simulink model "E_Platoon_simscape"  (R2025b)
settings: Solver=FixedStepAuto  StartTime=0.0  StopTime=inf  FixedStep=0.01  RelTol=1e-3
values from neighbouring files (symbols this model uses):
  battery_SOC_resistance = battery_SOC(:,3)    [EV_Truck.m]
  battery_SOC_SOC = battery_SOC(:,1)    [EV_Truck.m]
  battery_SOC_voltage = battery_SOC(:,2)    [EV_Truck.m]
  motor_efficiency_efficiency = table2array(motor_efficiency(2:height(motor_efficiency),2:width(motor_efficiency)))    [EV_Truck.m]
  motor_efficiency_RPM = table2array(motor_efficiency(2:height(motor_efficiency),1))    [EV_Truck.m]
  motor_efficiency_torque = transpose(motor_efficiency_torque)    [EV_Truck.m]
  motor_RPM_torque = table2array(motor_torque(1:14,1))    [EV_Truck.m]
  motor_torque_RPM = table2array(motor_torque(1:14,2))    [EV_Truck.m]
undefined symbols (not defined in the file or in its folder): battery_builder_rtmsupport, DiscIntNeverNeededParam, gcbh
libraries: simulink x8, fl_lib x8, nesl_utility x8, Batteries_lib x4, mpcadaslib x2, slpidlib x2
(part 2 of 3)

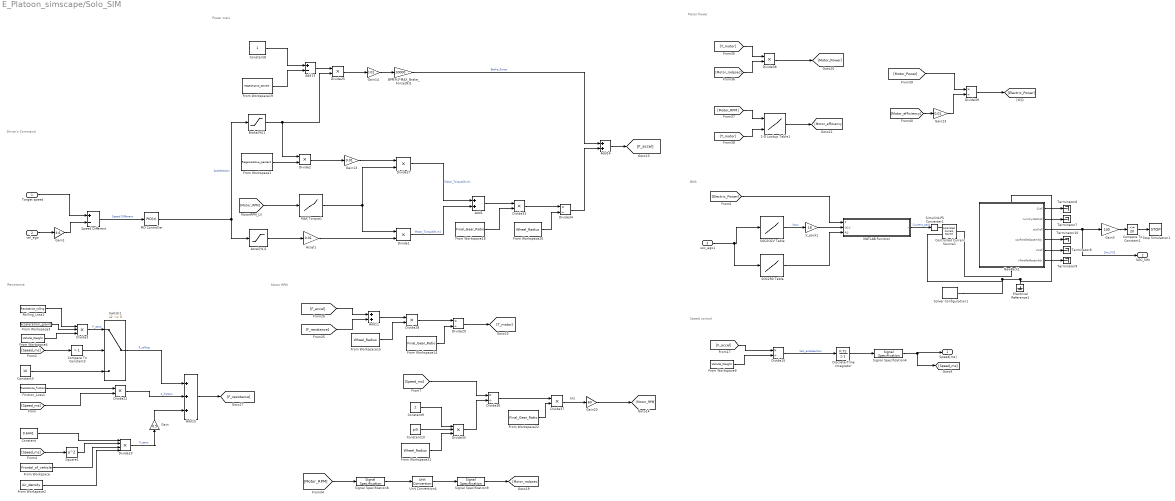
== system E_Platoon_simscape/Solo_SIM ==
  note: Speed control
  note: Driver's Command
  note: RPS
  note: Power train
  note: Resistance
  note: Motor RPM
  note: Motor Power
  note: BMS
  Target speed : Inport
  vel_ego : Inport  Port=2
  soc_ego1 : Inport  Port=3
  2-D Lookup Table1 : Lookup_n-D  BreakpointsForDimension1=motor_efficiency_RPM  BreakpointsForDimension2=motor_efficiency_torque  Table=motor_efficiency_efficiency  InternalRulePriority=Speed  RndMeth=Simplest
      settings: InputPortMap=u0,u1
  Accel1 : Gain  Gain=0.01
  Accel[%]1 : Saturate  UpperLimit=100  LowerLimit=0
  Add1 : Sum
  Add11 : Sum
  Add13 : Sum  Inputs=+-
  Add14 : Sum
  Add15 : Sum  Inputs=+++
  BPP[%]*MAX_Brake_Force[N]1 : Gain  Gain=10000
  Brake[%]1 : Saturate  UpperLimit=0  LowerLimit=-100
  Compare To Constant1 : simulink/Logic and Bit Operations/Compare To Constant  relop=<=  const=20  OutDataTypeStr=boolean
  Compare To Constant3 : simulink/Logic and Bit Operations/Compare To Constant  relop=>  const=1  OutDataTypeStr=boolean
  Constant : Constant  Value=0.6441
  Constant10 : Constant  Value=pi()
  Constant3 : Constant  Value=10
  Constant8 : Constant
  Constant9 : Constant  Value=2
  Controlled Current Source1 : fl_lib/Electrical/Electrical Sources/Controlled Current Source
  Discrete-Time Integrator : DiscreteIntegrator  SampleTime=-1  ICPrevOutput=DiscIntNeverNeededParam  ICPrevScaledInput=DiscIntNeverNeededParam
  Divide{1..2,22,25,27..28,33,37..38} (9 alike) : Product  Inputs=**
  Divide{15,29,34,36,39} (5 alike) : Product  Inputs=*/
  Divide23 : Product  Inputs=****
  Divide3 : Product  Inputs=***
  Divide35 : Product  Inputs=***
  Electrical Reference1 : fl_lib/Electrical/Electrical Elements/Electrical Reference
  Friction_Loss1 : FromWorkspace  VariableName=Resistance_friction  SampleTime=0.01
  From Workspace : FromWorkspace  VariableName=Frontal_of_vehicle  SampleTime=0.01
  From Workspace1 : FromWorkspace  VariableName=Regenerative_percent  SampleTime=0.01
  From Workspace14 : FromWorkspace  VariableName=Final_Gear_Ratio  SampleTime=0.01
  From Workspace15 : FromWorkspace  VariableName=Wheel_Radius  SampleTime=0.01
  From Workspace18 : FromWorkspace  VariableName=Final_Gear_Ratio  SampleTime=0.01
  From Workspace19 : FromWorkspace  VariableName=Regenerative_percent  SampleTime=0.01
  From Workspace2 : FromWorkspace  VariableName=Air_density  SampleTime=0.01
  From Workspace20 : FromWorkspace  VariableName=Wheel_Radius  SampleTime=0.01
  From Workspace21 : FromWorkspace  VariableName=Wheel_Radius  SampleTime=0.01
  From Workspace22 : FromWorkspace  VariableName=Final_Gear_Ratio  SampleTime=0.01
  From Workspace3 : FromWorkspace  VariableName=Acceleration_gravity  SampleTime=0.01
  From Workspace4 : FromWorkspace  VariableName=Vehicle_Weight  SampleTime=0.01
  From Workspace9 : FromWorkspace  VariableName=Vehicle_Weight  SampleTime=0.01
  Gain : Gain  Gain=0.5
  Gain1 : Gain  Gain=3.6
  Gain13 : Gain  Gain=0.01
  Gain14 : Gain  Gain=0.01
  Gain20 : Gain  Gain=60
  Gain23 : Gain  Gain=0.01
  Gain3 : Gain  Gain=100
  MATLAB Function : MATLAB Function  TreatAsAtomicUnit=on
  MAX Torque1 : Lookup_n-D  NumberOfTableDimensions=1  BreakpointsForDimension1=motor_RPM_torque  Table=motor_torque_RPM  InternalRulePriority=Speed  RndMeth=Simplest
  NewPack1 : Subsystem  LoadFcn=battery_builder_rtmsupport('loadfcn',gcbh);
      settings: CopyFcn=battery_builder_rtmsupport('copyfcn',gcbh);  PreCopyFcn=battery_builder_rtmsupport('precopyfcn',gcbh);  PreDeleteFcn=battery_builder_rtmsupport('predeletefcn',gcbh);  PortSchema="{\"entries\":[{\"content\":{\"sides\":[{\"content\":{\"connectorIds\":[\"LConn1\"]},\"type\":\"ConnectorPlacement.EquallySpacedRectSide\",\"uuid\":\"1202e0a0-be56-4819-949f-0e575ff0fad5\"},{\"content\":{\"connectorIds\":[\"RConn1\"],\"side\":\"RIGHT\"},\"type\":\"ConnectorPlacement.EquallySpacedRectSide\",\"uuid\":\"c846b010-7318-4529-a495-49262266c279\"},{\"content\":{\"side\":\"TOP\"},\"type\":\"ConnectorPlacement.EquallySpacedRectSide\",\"uuid\":\"5cadc0b8-a7f2-47b4-97e8-4fab1bc2ac7d\"},{\"content\":{\"connectorIds\":[\"Out1\",\"Out2\",\"Out3\",\"Out4\",\"Out5\",\"Out6\"],\"side\":\"BOTTOM\"},\"type\":\"ConnectorPlacement.EquallySpacedRectSide\",\"uuid\":\"c5ce92ef-d0c0-4ddc-9166-c3c67527b5cc\"}]},\"type\":\"ConnectorPlacement.EquallySpacedConnector\",\"uuid\":\"4d056c7c-5936-459e-9daf-456b1978dca2\"}],\"packageUris\":[\"http://schema.mathworks.com/mf0/Connector/R2020b\"],\"version\":\"1.0\"}"
      mask Display: image('$imagefile')
  PID Controller : slpidlib/PID Controller  Controller=PID  Form=Parallel  TimeDomain=Discrete-time  UseExternalTs=off  SampleTime=0.01  IntegratorMethod=Forward Euler  FilterMethod=Forward Euler  ControllerParametersSource=internal  P=100  I=0.01  UseKiTs=off  D=0.0001  UseExternalDerivativeSource=off  N=10  UseFilter=on  TunerSelectOption=Transfer Function Based (PID Tuner App)  InitialConditionSource=internal  InitialConditionForIntegrator=0  InitialConditionForFilter=0  DifferentiatorICPrevScaledInput=0  ExternalReset=none  TrackingMode=off  Kt=1  LimitOutput=off  SatLimitsSource=internal  UpperSaturationLimit=inf  LowerSaturationLimit=-inf  LinearizeAsGain=on  AntiWindupMode=none  Kb=1  LimitIntegrator=off  UpperIntegratorSaturationLimit=inf  LowerIntegratorSaturationLimit=-inf  POutMin=[]  POutMax=[]  IOutMin=[]  IOutMax=[]  DOutMin=[]  DOutMax=[]  NOutMin=[]  NOutMax=[]  SumOutMin=[]  SumOutMax=[]  SaturationOutMin=[]  SaturationOutMax=[]  PParamMin=[]  PParamMax=[]  IParamMin=[]  IParamMax=[]  DParamMin=[]  DParamMax=[]  NParamMin=[]  NParamMax=[]  KbParamMin=[]  KbParamMax=[]  KtParamMin=[]  KtParamMax=[]  KbOutMin=[]  KbOutMax=[]  KtOutMin=[]  KtOutMax=[]  IntegratorOutMin=[]  IntegratorOutMax=[]  FilterOutMin=[]  FilterOutMax=[]  SumI1OutMin=[]  SumI1OutMax=[]  SumI2OutMin=[]  SumI2OutMax=[]  SumI3OutMin=[]  SumI3OutMax=[]  SumI4OutMin=[]  SumI4OutMax=[]  SumDOutMin=[]  SumDOutMax=[]  DifferentiatorOutMin=[]  DifferentiatorOutMax=[]  FilterDiffOutCoefMin=[]  FilterDiffOutCoefMax=[]  ReciprocalOutMin=[]  ReciprocalOutMax=[]  SumDenOutMin=[]  SumDenOutMax=[]  SumNumOutMin=[]  SumNumOutMax=[]  DivideOutMin=[]  DivideOutMax=[]  UdiffTsProdOutMin=[]  UdiffTsProdOutMax=[]  NTsProdOutMin=[]  NTsProdOutMax=[]  UintegralTsProdOutMin=[]  UintegralTsProdOutMax=[]  UngainTsProdOutMin=[]  UngainTsProdOutMax=[]  ClampingZeroOutDataTypeStr=Inherit: Inherit via back propagation  ClampingZeroOutMin=[]  ClampingZeroOutMax=[]  FilterDenConstantOutDataTypeStr=Inherit: Inherit via back propagation  FilterDenConstantOutMin=[]  FilterDenConstantOutMax=[]  PCopyOutDataTypeStr=Inherit: Inherit via back propagation  PCopyOutMin=[]  PCopyOutMax=[]  NCopyOutDataTypeStr=Inherit: Inherit via back propagation  NCopyOutMin=[]  NCopyOutMax=[]  IntegratorContinuousStateAttributes=''  IntegratorStateMustResolveToSignalObject=off  IntegratorRTWStateStorageClass=Auto  FilterContinuousStateAttributes=''  FilterStateMustResolveToSignalObject=off  FilterRTWStateStorageClass=Auto  ParallelPVariant=InternalParameters  IdealPVariant=Disabled  IVariant=InternalParameters  DVariant=InternalParameters  IntegratorVariant=Discrete  SatVariant=Disabled  AWVariant=Passthrough  PCopyVariant=Disabled  TRVariant=Disabled  FdbkBlocksVariant=Forward  IdealPFdbkVariant=Disabled  SatFdbkVariant=Disabled  DerivativeFilterVariant=ForwardEulerFilter  NVariant=InternalParameters  NCopyVariant=Disabled  FilterICVariant=InternalICsFilter  IntegratorICVariant=InternalICs  ExternalResetVariant=Disabled  TRSumVariant=Passthrough  SumFdbkVariant=Disabled  SumVariant=Sum_PID  TsampFilterVariant=InternalTs  TsampNgainVariant=Passthrough  TsampIntegralVariant=Disabled_SignalSpec  ExternalSaturationOutDataTypeStr=Inherit: Same as second input  DerivativeSourceVariant=ErrorSignal  PreIntVariant=InternalPreInt
  Rolling_Loss1 : FromWorkspace  VariableName=Resistance_rolling  SampleTime=0.01
  SOC2OCV Table : Lookup_n-D  NumberOfTableDimensions=1  BreakpointsForDimension1=battery_SOC_SOC  Table=battery_SOC_voltage  ExtrapMethod=Clip  RemoveProtectionInput=on  UseLastTableValue=on  InternalRulePriority=Speed  RndMeth=Simplest
  SOC2R0 Table : Lookup_n-D  NumberOfTableDimensions=1  BreakpointsForDimension1=battery_SOC_SOC  Table=battery_SOC_resistance  RemoveProtectionInput=on  InternalRulePriority=Speed  RndMeth=Simplest
  Signal Specification4 : SignalSpecification  Unit=m/s
  Signal Specification8 : SignalSpecification  Unit=rpm
  Signal Specification9 : SignalSpecification  Unit=rad/s
  Simulink-PS Converter1 : nesl_utility/Simulink-PS Converter  PhysicalDomain=network_engine_domain  SubClassName=ps_input  LeftPortType=input  RightPortType=output  PseudoPeriodic=off  Frequencies=[]  NoiseDistribution=none  NoiseParameters=[]  Unit=1  AffineConversion=off  FilteringAndDerivatives=provide  SimscapeFilterOrder=1  InputFilterTimeConstant=0.001  UdotUserProvided=0
  Solver Configuration1 : nesl_utility/Solver Configuration  PhysicalDomain=network_engine_domain  SubClassName=solver  LeftPortType=input  RightPortType=generic  Tones=[]  Harmonics=[]  SimulateNoise=off  Profile=off  UseLocalSampling=off  EnableSwitchedLinearOptims=on  FrequencyDomain=off  UseCCode=off  RelTol=0.001  AbsTol=0.001  MinStep=1e-09  ToWorkspace=off  RevertToSquareIcSolve=off  NumHomotopyIterations=100  PhasorMode=off  PhasorModeNumHarmonics=1  ConsistencySolver=NEWTON_XTOL_AFTER_FTOL  IndexReductionMethod=DerivativeReplacement  DoDC=on  ResidualTolerance=1e-09  ConsistencyTolSource=GLOBAL  ConsistencyAbsTol=0.001  ConsistencyRelTol=0.001  ConsistencyTolFactor=0.001  UseLocalSolver=off  LocalSolverChoice=NE_BACKWARD_EULER_ADVANCER  ResolveIndetEquations=on  FunctionEvalNumThread=1  LocalSolverSampleTime=0.01  DoFixedCost=off  MaxNonlinIter=3  MaxModeIter=2  ComputeImpulses=off  ImpulseIterations=2  LinearAlgebra=auto  LinearAlgebraNumThread=0  EquationFormulation=NE_TIME_EF  DelaysMemoryBudget=1024  AutomaticFiltering=on  FilteringTimeConstant=0.001  PartitionStorageMethod=AS_NEEDED  PartitionMemoryBudget=1024  PartitionMethod=ROBUST  MultibodyUseLocalSolver=off  MultibodyLocalSolverChoice=ODE1  MultibodyLocalSolverSampleTime=0.001
  Speed Different : Sum  Inputs=+-
  Square1 : Math  Operator=square
  Stop Simulation1 : Stop
  Switch1 : Switch  Criteria=u2 ~= 0  SaturateOnIntegerOverflow=off  InputSameDT=off
  Terminator{6..10} (5 alike) : Terminator
  Unit Conversion4 : UnitConversion
  V_pack1 : Gain  Gain=18
  Speed[ms] : Outport
  SOC_SIM : Outport  Port=2
  wires:
  From Workspace9/1 -> Divide15/2
  Divide15/1 -> Discrete-Time Integrator/1  "Veh_acceleartion"
  Discrete-Time Integrator/1 -> Signal Specification4/1
  Signal Specification4/1 -> Speed[ms]/1, [Speed_ms]
  PID Controller/1 -> Brake[%]1/1, Accel[%]1/1  "Acceleration"
  Speed Different/1 -> PID Controller/1  "Speed Different"
  Target speed/1 -> Speed Different/1
  vel_ego/1 -> Gain1/1
  Divide28/1 -> Divide29/1
  From Workspace20/1 -> Divide34/2
  Add1/1 -> Divide33/1
  [T_motor] -> Divide38/1
  Divide29/1 -> [T_motor]
  Signal Specification9/1 -> [Motor_radpsec]
  Gain20/1 -> [Motor_RPM]
  Add13/1 -> Divide25/1
  Divide39/1 -> [Electric_Power]
  Add14/1 -> [F_accel]
  [Speed_ms] -> Divide22/2
  [F_resistance] -> Add11/2
  Divide1/1 -> Add1/2  "Motor_Torque[N.m]"
  From Workspace14/1 -> Divide29/2
  Divide23/1 -> Gain/1  "F_aero"
  Brake[%]1/1 -> Divide25/2, Divide2/1
  Unit Conversion4/1 -> Signal Specification9/1
  From Workspace21/1 -> Divide35/3
  Divide35/1 -> Divide36/2
  [Motor_RPM] -> 2-D Lookup Table1/1
  Gain23/1 -> Divide39/2
  Compare To Constant3/1 -> Switch1/2
  Divide37/1 -> Gain20/1
  Divide34/1 -> Add14/2
  BPP[%]*MAX_Brake_Force[N]1/1 -> Add14/1  "Brake_Force"
  From Workspace/1 -> Divide23/3
  From Workspace22/1 -> Divide37/2
  Constant9/1 -> Divide35/1
  [Motor_efficiency] -> Gain23/1
  Constant10/1 -> Divide35/2
  [Speed_ms] -> Square1/1
  Add11/1 -> Divide28/1
  Square1/1 -> Divide23/2
  2-D Lookup Table1/1 -> [Motor_efficiency]
  Gain14/1 -> BPP[%]*MAX_Brake_Force[N]1/1
  From Workspace19/1 -> Add13/2
  Add15/1 -> [F_resistance]
  Friction_Loss1/1 -> Divide22/1
  [Motor_RPM] -> Signal Specification8/1
  [Motor_radpsec] -> Divide38/2
  From Workspace1/1 -> Divide2/2
  Accel[%]1/1 -> Accel1/1
  Constant8/1 -> Add13/1
  Divide36/1 -> Divide37/1
  [Motor_Power] -> Divide39/1
  MAX Torque1/1 -> Divide27/2, Divide1/1
  Accel1/1 -> Divide1/2
  Divide33/1 -> Divide34/1
  [F_accel] -> Add11/1
  [T_motor] -> 2-D Lookup Table1/2
  Rolling_Loss1/1 -> Divide3/1
  Divide27/1 -> Add1/1  "Motor_Torque[N.m]"
  Switch1/1 -> Add15/1  "F_rolling"
  From Workspace15/1 -> Divide28/2
  Gain13/1 -> Divide27/1
  Constant3/1 -> Switch1/3
  Divide25/1 -> Gain14/1
  Divide22/1 -> Add15/2  "F_friction"
  Divide2/1 -> Gain13/1
  Divide38/1 -> [Motor_Power]
  [Motor_RPM] -> MAX Torque1/1
  Signal Specification8/1 -> Unit Conversion4/1
  From Workspace18/1 -> Divide33/2
  [Speed_ms] -> Divide36/1
  [F_accel] -> Divide15/1
  [Speed_ms] -> Compare To Constant3/1
  Gain/1 -> Add15/3
  From Workspace2/1 -> Divide23/4
  From Workspace3/1 -> Divide3/2
  From Workspace4/1 -> Divide3/3
  Divide3/1 -> Switch1/1  "F_aero"
  Gain1/1 -> Speed Different/2
  Constant/1 -> Divide23/1
  SOC2R0 Table/1 -> MATLAB Function/3(R0)
  MATLAB Function/1(I) -> Simulink-PS Converter1/1  "Current_pack"
  Compare To Constant1/1 -> Stop Simulation1/1
  soc_ego1/1 -> SOC2R0 Table/1, SOC2OCV Table/1
  [Electric_Power] -> MATLAB Function/1(P)
  NewPack1/6(vParallelAssembly) -> Terminator9/1
  NewPack1/4(socParallelAssembly) -> Terminator10/1
  NewPack1/3(socCell) -> SOC_SIM/1, Gain3/1  "Sim_FV2"
  V_pack1/1 -> MATLAB Function/2(OCV)
  NewPack1/2(numCyclesCell) -> Terminator7/1
  SOC2OCV Table/1 -> V_pack1/1  "Vsoc"
  NewPack1/1(iCell) -> Terminator6/1
  NewPack1/5(vCell) -> Terminator8/1
  Gain3/1 -> Compare To Constant1/1
  connections:
  Electrical Reference1/LConn1 -- NewPack1/LConn1 -- Controlled Current Source1/RConn2 -- Solver Configuration1/RConn1
  NewPack1/RConn1 -- Controlled Current Source1/LConn1
  Simulink-PS Converter1/RConn1 -- Controlled Current Source1/RConn1

== system E_Platoon_simscape/FV1_SIM/ACC system ==
  vel_front : Inport
  pos_front : Inport  Port=2
  vel_ego : Inport  Port=3
  pos_ego : Inport  Port=4
  Adaptive Cruise Control System : mpcadaslib/Adaptive Cruise Control System  EgoModel=tf(1,[0.5,1,0])  InitialEgoVelocity=20  DefaultSpacing=20  MaxVelocity=30  MinAcceleration=-3  amin_ext=off  MaxAcceleration=3  amax_ext=off  Ts=0.01  PredictionHorizon=100  ControllerBehavior=0.7  suboptimal=off  maxiter=10  datatypeopt=double  optmode=off  trackmode=off
  MATLAB Function : MATLAB Function  TreatAsAtomicUnit=on
  Sum : Sum  Inputs=|+-
  Sum1 : Sum  Inputs=|-+
  t_gap(s) : Constant  Value=0.5
  velocity(m/s) : Constant  Value=30
  Acceleration : Outport
  Relative Distance : Outport  Port=2
  wires:
  t_gap(s)/1 -> Adaptive Cruise Control System/2
  Sum/1 -> Relative Distance/1, Adaptive Cruise Control System/4
  Sum1/1 -> Adaptive Cruise Control System/5
  velocity(m/s)/1 -> Adaptive Cruise Control System/1
  Adaptive Cruise Control System/1 -> MATLAB Function/1(accel)
  pos_front/1 -> Sum/1
  pos_ego/1 -> Sum/2
  vel_front/1 -> Sum1/2
  vel_ego/1 -> Sum1/1, Adaptive Cruise Control System/3
  MATLAB Function/1(acceleration) -> Acceleration/1

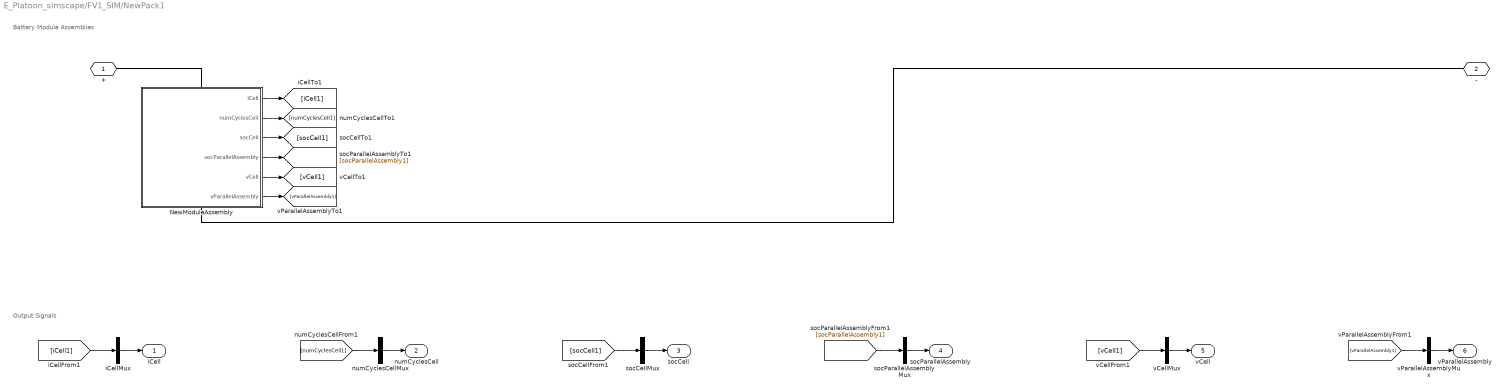
== system E_Platoon_simscape/FV1_SIM/NewPack1 ==
  note: Battery Module Assemblies
  note: Output Signals
  NewModuleAssembly : Subsystem  LoadFcn=battery_builder_rtmsupport('loadfcn',gcbh);
      settings: CopyFcn=battery_builder_rtmsupport('copyfcn',gcbh);  PreCopyFcn=battery_builder_rtmsupport('precopyfcn',gcbh);  PreDeleteFcn=battery_builder_rtmsupport('predeletefcn',gcbh);  PortSchema="{\"entries\":[{\"content\":{\"sides\":[{\"content\":{\"connectorIds\":[\"LConn1\"]},\"type\":\"ConnectorPlacement.EquallySpacedRectSide\",\"uuid\":\"1202e0a0-be56-4819-949f-0e575ff0fad5\"},{\"content\":{\"connectorIds\":[\"RConn1\"],\"side\":\"RIGHT\"},\"type\":\"ConnectorPlacement.EquallySpacedRectSide\",\"uuid\":\"c846b010-7318-4529-a495-49262266c279\"},{\"content\":{\"side\":\"TOP\"},\"type\":\"ConnectorPlacement.EquallySpacedRectSide\",\"uuid\":\"5cadc0b8-a7f2-47b4-97e8-4fab1bc2ac7d\"},{\"content\":{\"connectorIds\":[\"Out1\",\"Out2\",\"Out3\",\"Out4\",\"Out5\",\"Out6\"],\"side\":\"BOTTOM\"},\"type\":\"ConnectorPlacement.EquallySpacedRectSide\",\"uuid\":\"9f2ef959-f133-4a8d-a7c5-293375a4069f\"}]},\"type\":\"ConnectorPlacement.EquallySpacedConnector\",\"uuid\":\"4d056c7c-5936-459e-9daf-456b1978dca2\"}],\"packageUris\":[\"http://schema.mathworks.com/mf0/Connector/R2020b\"],\"version\":\"1.0\"}"
      mask Display: image('$imagefile')
  iCellMux : Mux  Inputs=1
  numCyclesCellMux : Mux  Inputs=1
  socCellMux : Mux  Inputs=1
  socParallelAssemblyMux : Mux  Inputs=1
  vCellMux : Mux  Inputs=1
  vParallelAssemblyMux : Mux  Inputs=1
  + : PMIOPort  Side=Left
  - : PMIOPort  Port=2  Side=Right
  iCell : Outport
  numCyclesCell : Outport  Port=2
  socCell : Outport  Port=3
  socParallelAssembly : Outport  Port=4
  vCell : Outport  Port=5
  vParallelAssembly : Outport  Port=6
  wires:
  NewModuleAssembly/1(iCell) -> [iCell1]
  iCellMux/1 -> iCell/1
  [iCell1] -> iCellMux/1
  NewModuleAssembly/2(numCyclesCell) -> [numCyclesCell1]
  numCyclesCellMux/1 -> numCyclesCell/1
  [numCyclesCell1] -> numCyclesCellMux/1
  NewModuleAssembly/3(socCell) -> [socCell1]
  socCellMux/1 -> socCell/1
  [socCell1] -> socCellMux/1
  NewModuleAssembly/4(socParallelAssembly) -> [socParallelAssembly1]
  socParallelAssemblyMux/1 -> socParallelAssembly/1
  [socParallelAssembly1] -> socParallelAssemblyMux/1
  NewModuleAssembly/5(vCell) -> [vCell1]
  vCellMux/1 -> vCell/1
  [vCell1] -> vCellMux/1
  NewModuleAssembly/6(vParallelAssembly) -> [vParallelAssembly1]
  vParallelAssemblyMux/1 -> vParallelAssembly/1
  [vParallelAssembly1] -> vParallelAssemblyMux/1
  connections:
  NewModuleAssembly/LConn1 -- +/RConn1
  NewModuleAssembly/RConn1 -- -/RConn1

== system E_Platoon_simscape/FV2_SIM/ACC system ==
  vel_front : Inport
  pos_front : Inport  Port=2
  vel_ego : Inport  Port=3
  pos_ego : Inport  Port=4
  Adaptive Cruise Control System : mpcadaslib/Adaptive Cruise Control System  EgoModel=tf(1,[0.5,1,0])  InitialEgoVelocity=20  DefaultSpacing=20  MaxVelocity=30  MinAcceleration=-3  amin_ext=off  MaxAcceleration=3  amax_ext=off  Ts=0.01  PredictionHorizon=100  ControllerBehavior=0.7  suboptimal=off  maxiter=10  datatypeopt=double  optmode=off  trackmode=off
  MATLAB Function : MATLAB Function  TreatAsAtomicUnit=on
  Sum : Sum  Inputs=|+-
  Sum1 : Sum  Inputs=|-+
  t_gap(s) : Constant  Value=0.5
  velocity(m/s) : Constant  Value=30
  Acceleration : Outport
  Relative Distance : Outport  Port=2
  wires:
  t_gap(s)/1 -> Adaptive Cruise Control System/2
  Sum/1 -> Relative Distance/1, Adaptive Cruise Control System/4
  Sum1/1 -> Adaptive Cruise Control System/5
  velocity(m/s)/1 -> Adaptive Cruise Control System/1
  Adaptive Cruise Control System/1 -> MATLAB Function/1(accel)
  pos_front/1 -> Sum/1
  pos_ego/1 -> Sum/2
  vel_front/1 -> Sum1/2
  vel_ego/1 -> Sum1/1, Adaptive Cruise Control System/3
  MATLAB Function/1(acceleration) -> Acceleration/1

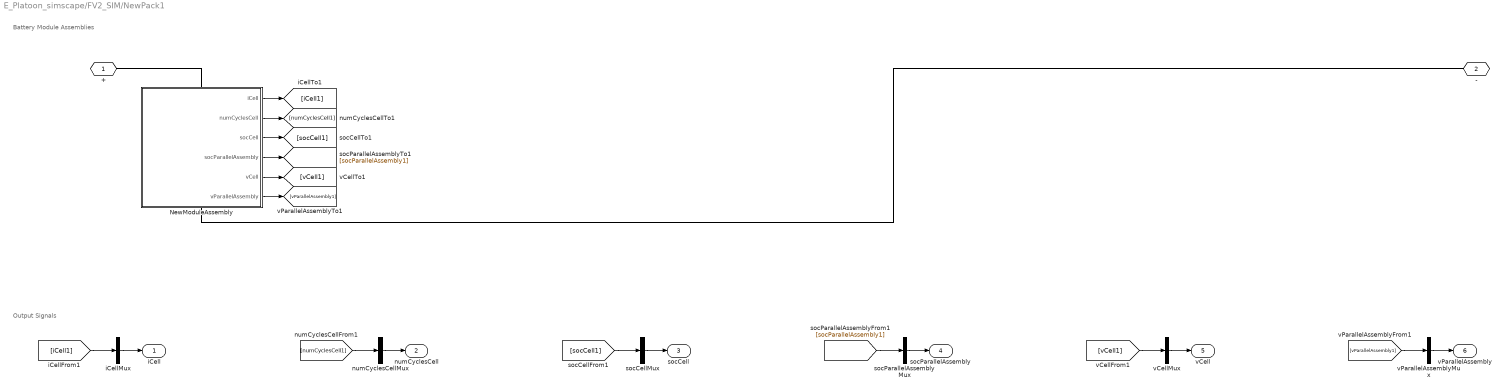
== system E_Platoon_simscape/FV2_SIM/NewPack1 ==
  note: Battery Module Assemblies
  note: Output Signals
  NewModuleAssembly : Subsystem  LoadFcn=battery_builder_rtmsupport('loadfcn',gcbh);
      settings: CopyFcn=battery_builder_rtmsupport('copyfcn',gcbh);  PreCopyFcn=battery_builder_rtmsupport('precopyfcn',gcbh);  PreDeleteFcn=battery_builder_rtmsupport('predeletefcn',gcbh);  PortSchema="{\"entries\":[{\"content\":{\"sides\":[{\"content\":{\"connectorIds\":[\"LConn1\"]},\"type\":\"ConnectorPlacement.EquallySpacedRectSide\",\"uuid\":\"1202e0a0-be56-4819-949f-0e575ff0fad5\"},{\"content\":{\"connectorIds\":[\"RConn1\"],\"side\":\"RIGHT\"},\"type\":\"ConnectorPlacement.EquallySpacedRectSide\",\"uuid\":\"c846b010-7318-4529-a495-49262266c279\"},{\"content\":{\"side\":\"TOP\"},\"type\":\"ConnectorPlacement.EquallySpacedRectSide\",\"uuid\":\"5cadc0b8-a7f2-47b4-97e8-4fab1bc2ac7d\"},{\"content\":{\"connectorIds\":[\"Out1\",\"Out2\",\"Out3\",\"Out4\",\"Out5\",\"Out6\"],\"side\":\"BOTTOM\"},\"type\":\"ConnectorPlacement.EquallySpacedRectSide\",\"uuid\":\"9f2ef959-f133-4a8d-a7c5-293375a4069f\"}]},\"type\":\"ConnectorPlacement.EquallySpacedConnector\",\"uuid\":\"4d056c7c-5936-459e-9daf-456b1978dca2\"}],\"packageUris\":[\"http://schema.mathworks.com/mf0/Connector/R2020b\"],\"version\":\"1.0\"}"
      mask Display: image('$imagefile')
  iCellMux : Mux  Inputs=1
  numCyclesCellMux : Mux  Inputs=1
  socCellMux : Mux  Inputs=1
  socParallelAssemblyMux : Mux  Inputs=1
  vCellMux : Mux  Inputs=1
  vParallelAssemblyMux : Mux  Inputs=1
  + : PMIOPort  Side=Left
  - : PMIOPort  Port=2  Side=Right
  iCell : Outport
  numCyclesCell : Outport  Port=2
  socCell : Outport  Port=3
  socParallelAssembly : Outport  Port=4
  vCell : Outport  Port=5
  vParallelAssembly : Outport  Port=6
  wires:
  NewModuleAssembly/1(iCell) -> [iCell1]
  iCellMux/1 -> iCell/1
  [iCell1] -> iCellMux/1
  NewModuleAssembly/2(numCyclesCell) -> [numCyclesCell1]
  numCyclesCellMux/1 -> numCyclesCell/1
  [numCyclesCell1] -> numCyclesCellMux/1
  NewModuleAssembly/3(socCell) -> [socCell1]
  socCellMux/1 -> socCell/1
  [socCell1] -> socCellMux/1
  NewModuleAssembly/4(socParallelAssembly) -> [socParallelAssembly1]
  socParallelAssemblyMux/1 -> socParallelAssembly/1
  [socParallelAssembly1] -> socParallelAssemblyMux/1
  NewModuleAssembly/5(vCell) -> [vCell1]
  vCellMux/1 -> vCell/1
  [vCell1] -> vCellMux/1
  NewModuleAssembly/6(vParallelAssembly) -> [vParallelAssembly1]
  vParallelAssemblyMux/1 -> vParallelAssembly/1
  [vParallelAssembly1] -> vParallelAssemblyMux/1
  connections:
  NewModuleAssembly/LConn1 -- +/RConn1
  NewModuleAssembly/RConn1 -- -/RConn1

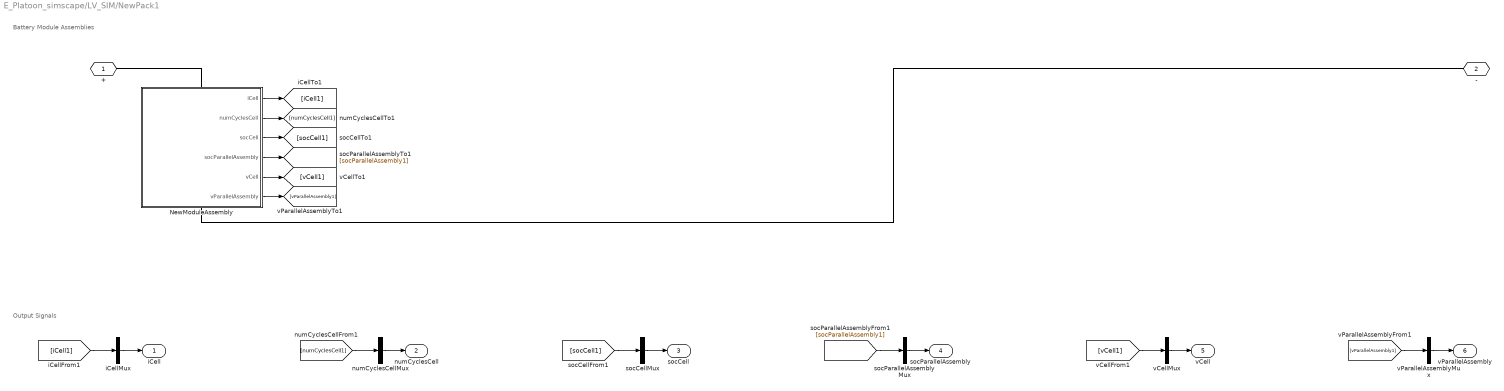
== system E_Platoon_simscape/LV_SIM/NewPack1 ==
  note: Battery Module Assemblies
  note: Output Signals
  NewModuleAssembly : Subsystem  LoadFcn=battery_builder_rtmsupport('loadfcn',gcbh);
      settings: CopyFcn=battery_builder_rtmsupport('copyfcn',gcbh);  PreCopyFcn=battery_builder_rtmsupport('precopyfcn',gcbh);  PreDeleteFcn=battery_builder_rtmsupport('predeletefcn',gcbh);  PortSchema="{\"entries\":[{\"content\":{\"sides\":[{\"content\":{\"connectorIds\":[\"LConn1\"]},\"type\":\"ConnectorPlacement.EquallySpacedRectSide\",\"uuid\":\"1202e0a0-be56-4819-949f-0e575ff0fad5\"},{\"content\":{\"connectorIds\":[\"RConn1\"],\"side\":\"RIGHT\"},\"type\":\"ConnectorPlacement.EquallySpacedRectSide\",\"uuid\":\"c846b010-7318-4529-a495-49262266c279\"},{\"content\":{\"side\":\"TOP\"},\"type\":\"ConnectorPlacement.EquallySpacedRectSide\",\"uuid\":\"5cadc0b8-a7f2-47b4-97e8-4fab1bc2ac7d\"},{\"content\":{\"connectorIds\":[\"Out1\",\"Out2\",\"Out3\",\"Out4\",\"Out5\",\"Out6\"],\"side\":\"BOTTOM\"},\"type\":\"ConnectorPlacement.EquallySpacedRectSide\",\"uuid\":\"9f2ef959-f133-4a8d-a7c5-293375a4069f\"}]},\"type\":\"ConnectorPlacement.EquallySpacedConnector\",\"uuid\":\"4d056c7c-5936-459e-9daf-456b1978dca2\"}],\"packageUris\":[\"http://schema.mathworks.com/mf0/Connector/R2020b\"],\"version\":\"1.0\"}"
      mask Display: image('$imagefile')
  iCellMux : Mux  Inputs=1
  numCyclesCellMux : Mux  Inputs=1
  socCellMux : Mux  Inputs=1
  socParallelAssemblyMux : Mux  Inputs=1
  vCellMux : Mux  Inputs=1
  vParallelAssemblyMux : Mux  Inputs=1
  + : PMIOPort  Side=Left
  - : PMIOPort  Port=2  Side=Right
  iCell : Outport
  numCyclesCell : Outport  Port=2
  socCell : Outport  Port=3
  socParallelAssembly : Outport  Port=4
  vCell : Outport  Port=5
  vParallelAssembly : Outport  Port=6
  wires:
  NewModuleAssembly/1(iCell) -> [iCell1]
  iCellMux/1 -> iCell/1
  [iCell1] -> iCellMux/1
  NewModuleAssembly/2(numCyclesCell) -> [numCyclesCell1]
  numCyclesCellMux/1 -> numCyclesCell/1
  [numCyclesCell1] -> numCyclesCellMux/1
  NewModuleAssembly/3(socCell) -> [socCell1]
  socCellMux/1 -> socCell/1
  [socCell1] -> socCellMux/1
  NewModuleAssembly/4(socParallelAssembly) -> [socParallelAssembly1]
  socParallelAssemblyMux/1 -> socParallelAssembly/1
  [socParallelAssembly1] -> socParallelAssemblyMux/1
  NewModuleAssembly/5(vCell) -> [vCell1]
  vCellMux/1 -> vCell/1
  [vCell1] -> vCellMux/1
  NewModuleAssembly/6(vParallelAssembly) -> [vParallelAssembly1]
  vParallelAssemblyMux/1 -> vParallelAssembly/1
  [vParallelAssembly1] -> vParallelAssemblyMux/1
  connections:
  NewModuleAssembly/LConn1 -- +/RConn1
  NewModuleAssembly/RConn1 -- -/RConn1

== system E_Platoon_simscape/Solo_SIM/NewPack1 ==
  note: Battery Module Assemblies
  note: Output Signals
  NewModuleAssembly : Subsystem  LoadFcn=battery_builder_rtmsupport('loadfcn',gcbh);
      settings: CopyFcn=battery_builder_rtmsupport('copyfcn',gcbh);  PreCopyFcn=battery_builder_rtmsupport('precopyfcn',gcbh);  PreDeleteFcn=battery_builder_rtmsupport('predeletefcn',gcbh);  PortSchema="{\"entries\":[{\"content\":{\"sides\":[{\"content\":{\"connectorIds\":[\"LConn1\"]},\"type\":\"ConnectorPlacement.EquallySpacedRectSide\",\"uuid\":\"1202e0a0-be56-4819-949f-0e575ff0fad5\"},{\"content\":{\"connectorIds\":[\"RConn1\"],\"side\":\"RIGHT\"},\"type\":\"ConnectorPlacement.EquallySpacedRectSide\",\"uuid\":\"c846b010-7318-4529-a495-49262266c279\"},{\"content\":{\"side\":\"TOP\"},\"type\":\"ConnectorPlacement.EquallySpacedRectSide\",\"uuid\":\"5cadc0b8-a7f2-47b4-97e8-4fab1bc2ac7d\"},{\"content\":{\"connectorIds\":[\"Out1\",\"Out2\",\"Out3\",\"Out4\",\"Out5\",\"Out6\"],\"side\":\"BOTTOM\"},\"type\":\"ConnectorPlacement.EquallySpacedRectSide\",\"uuid\":\"9f2ef959-f133-4a8d-a7c5-293375a4069f\"}]},\"type\":\"ConnectorPlacement.EquallySpacedConnector\",\"uuid\":\"4d056c7c-5936-459e-9daf-456b1978dca2\"}],\"packageUris\":[\"http://schema.mathworks.com/mf0/Connector/R2020b\"],\"version\":\"1.0\"}"
      mask Display: image('$imagefile')
  iCellMux : Mux  Inputs=1
  numCyclesCellMux : Mux  Inputs=1
  socCellMux : Mux  Inputs=1
  socParallelAssemblyMux : Mux  Inputs=1
  vCellMux : Mux  Inputs=1
  vParallelAssemblyMux : Mux  Inputs=1
  + : PMIOPort  Side=Left
  - : PMIOPort  Port=2  Side=Right
  iCell : Outport
  numCyclesCell : Outport  Port=2
  socCell : Outport  Port=3
  socParallelAssembly : Outport  Port=4
  vCell : Outport  Port=5
  vParallelAssembly : Outport  Port=6
  wires:
  NewModuleAssembly/1(iCell) -> [iCell1]
  iCellMux/1 -> iCell/1
  [iCell1] -> iCellMux/1
  NewModuleAssembly/2(numCyclesCell) -> [numCyclesCell1]
  numCyclesCellMux/1 -> numCyclesCell/1
  [numCyclesCell1] -> numCyclesCellMux/1
  NewModuleAssembly/3(socCell) -> [socCell1]
  socCellMux/1 -> socCell/1
  [socCell1] -> socCellMux/1
  NewModuleAssembly/4(socParallelAssembly) -> [socParallelAssembly1]
  socParallelAssemblyMux/1 -> socParallelAssembly/1
  [socParallelAssembly1] -> socParallelAssemblyMux/1
  NewModuleAssembly/5(vCell) -> [vCell1]
  vCellMux/1 -> vCell/1
  [vCell1] -> vCellMux/1
  NewModuleAssembly/6(vParallelAssembly) -> [vParallelAssembly1]
  vParallelAssemblyMux/1 -> vParallelAssembly/1
  [vParallelAssembly1] -> vParallelAssemblyMux/1
  connections:
  NewModuleAssembly/LConn1 -- +/RConn1
  NewModuleAssembly/RConn1 -- -/RConn1

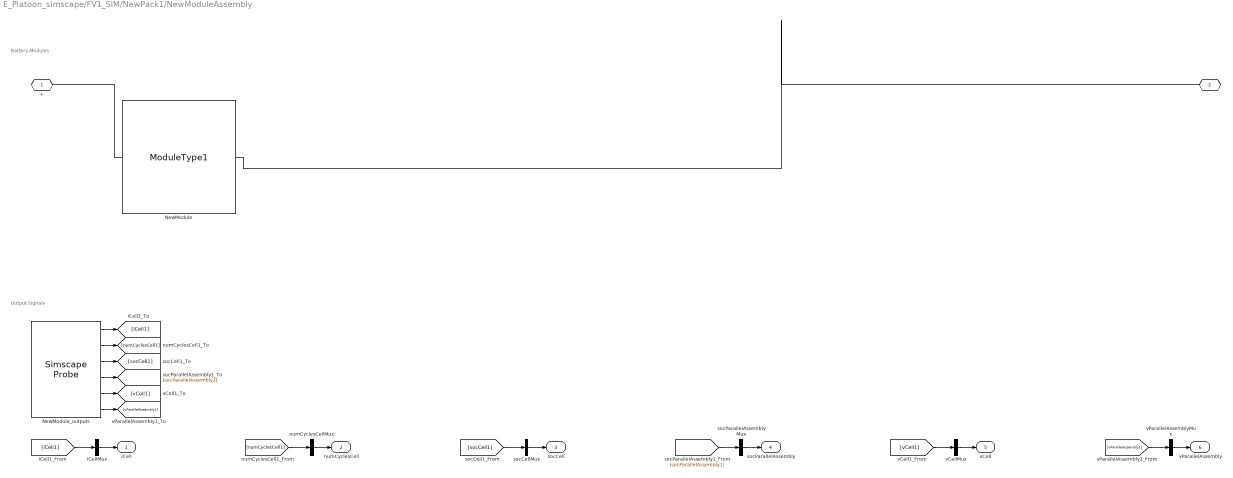
== system E_Platoon_simscape/FV1_SIM/NewPack1/NewModuleAssembly ==
  note: Output Signals
  note: Battery Modules
  NewModule : Batteries_lib/Modules/ModuleType1  SOC_vecCell=[0, .01, .02, .03, .04, .05, .06, .07, .08, .09, .1, .11, .12, .13, .14, .15, .16, .17, .18, .19, .2, .21, .22, .23, .24, .25, .26, .27, .28, .29, .3, .31, .32, .33, .34, .35, .36, .37, .38, .39, .4, .41, .42, .43, .44, .45, .46, .47, .48, .49, .5, .51, .52, .53, .54, .55, .56, .57, .58, .59, .6, .61, .62, .63, .64, .65, .66, .67, .68, .69, .7, .71, .72, .73, .74, .75, .76, .77, .78, .79, .8, .81, .82, .83, .84, .85, .86, .87, .88, .89, .9, .91, .92, .93, .94, .95, .96, .97, .98, .99, 1]  V0_vecCell=[35.84591, 36.10202, 36.35814, 36.61425, 36.87037, 37.12649, 37.3826, 37.63872, 37.89483, 38.09951, 38.20904, 38.28916, 38.37306, 38.42308, 38.45482, 38.47744, 38.49779, 38.54815, 38.5883, 38.63829, 38.68732, 38.72975, 38.77111, 38.80795, 38.83724, 38.8617, 38.89023, 38.9273, 38.96054, 38.98786, 39.01519, 39.03864, 39.06385, 39.08223, 39.1006, 39.11898, 39.13735, 39.15508, 39.16412, 39.17437, 39.18528, 39.19619, 39.20709, 39.21696, 39.22232, 39.22753, 39.23277, 39.23672, 39.23942, 39.24211, 39.24481, 39.24786, 39.25094, 39.2539, 39.25686, 39.26099, 39.26708, 39.27551, 39.28394, 39.29233, 39.30067, 39.31557, 39.33487, 39.35402, 39.37113, 39.38825, 39.40815, 39.43406, 39.46187, 39.48968, 39.51913, 39.55031, 39.5817, 39.60619, 39.62271, 39.63907, 39.65521, 39.67134, 39.68137, 39.69071, 39.70005, 39.7052, 39.70868, 39.70916, 39.70862, 39.70807, 39.70752, 39.71037, 39.72142, 39.72908, 39.73651, 39.73911, 39.73577, 39.72919, 39.73278, 39.7392, 39.74638, 39.75462, 39.8136, 40.01141, 40.30627] V  V_rangeCell=[27, Inf] V  R0_vecCell=[.47635, .41138, .35007, .29417, .24882, .2142, .18886, .17031, .1569, .14398, .13028, .11716, .10632, .09512, .08414, .07347, .06467, .05964, .05477, .05154, .04841, .04625, .04448, .04297, .04112, .03908, .0378, .03771, .03746, .03699, .03652, .03598, .03587, .03552, .03517, .03481, .03446, .03417, .03358, .03336, .03321, .03305, .0329, .0327, .03227, .03186, .03148, .03105, .03058, .03011, .02964, .02918, .02875, .02834, .02792, .02762, .02745, .02737, .02729, .02722, .02715, .0274, .02786, .0283, .02854, .02877, .02906, .02956, .03013, .0307, .03135, .03204, .03271, .03308, .03307, .03314, .03323, .03332, .03312, .03288, .03264, .03224, .03172, .03113, .03057, .03001, .02945, .02905, .02924, .0293, .02938, .02923, .02879, .02803, .02792, .02793, .02786, .02652, .02587, .02701, .00941] Ohm  AHCell=50.41 A*hr  extrapolation_optionCell=simscape.enum.extrapolation.nearest  P=18  S=18  iCell_specify=off  iCell_priority=None  iCell=0 A  iCell_nominal_specify=off  iCell_nominal_value=1  iCell_nominal_unit=A  vCell_specify=off  vCell_priority=None  vCell=0 V  vCell_nominal_specify=off  vCell_nominal_value=1  vCell_nominal_unit=V  socCell_specify=off  socCell_priority=High  socCell=1  socCell_nominal_specify=off  socCell_nominal_value=1  socCell_nominal_unit=1  numCyclesCell_specify=off  numCyclesCell_priority=High  numCyclesCell=0  numCyclesCell_nominal_specify=off  numCyclesCell_nominal_value=1  numCyclesCell_nominal_unit=1  vParallelAssembly_specify=off  vParallelAssembly_priority=None  vParallelAssembly=repmat(0, 18, 1) V  vParallelAssembly_nominal_specify=off  vParallelAssembly_nominal_value=1  vParallelAssembly_nominal_unit=V  socParallelAssembly_specify=off  socParallelAssembly_priority=None  socParallelAssembly=repmat(1, 18, 1)  socParallelAssembly_nominal_specify=off  socParallelAssembly_nominal_value=1  socParallelAssembly_nominal_unit=1
      settings: InternalSimscapePortConfiguration="{\"Bottom\":[{\"id\":\"n\",\"label\":\"-\",\"type\":\"foundation.electrical.electrical\"}],\"Left\":[],\"Right\":[],\"Top\":[{\"id\":\"p\",\"label\":\"+\",\"type\":\"foundation.electrical.electrical\"}]}"
  NewModule_outputs : SimscapeProbe  BoundBlock=11139  Variables="{\"iCell\":{\"Unit\":\"A\",\"PortLabel\":\"iCell\",\"Probing\":\"ON\"},\"numCyclesCell\":{\"Unit\":\"1\",\"PortLabel\":\"numCyclesCell\",\"Probing\":\"ON\"},\"socCell\":{\"Unit\":\"1\",\"PortLabel\":\"socCell\",\"Probing\":\"ON\"},\"socParallelAssembly\":{\"Unit\":\"1\",\"PortLabel\":\"socParallelAssembly\",\"Probing\":\"ON\"},\"vCell\":{\"Unit\":\"V\",\"PortLabel\":\"vCell\",\"Probing\":\"ON\"},\"vParallelAssembly\":{\"Unit\":\"V\",\"PortLabel\":\"vParallelAssembly\",\"Probing\":\"ON\"}}"
  iCellMux : Mux  Inputs=1
  numCyclesCellMux : Mux  Inputs=1
  socCellMux : Mux  Inputs=1
  socParallelAssemblyMux : Mux  Inputs=1
  vCellMux : Mux  Inputs=1
  vParallelAssemblyMux : Mux  Inputs=1
  + : PMIOPort  Side=Left
  - : PMIOPort  Port=2  Side=Right
  iCell : Outport
  numCyclesCell : Outport  Port=2
  socCell : Outport  Port=3
  socParallelAssembly : Outport  Port=4
  vCell : Outport  Port=5
  vParallelAssembly : Outport  Port=6
  wires:
  [vParallelAssembly1] -> vParallelAssemblyMux/1
  vParallelAssemblyMux/1 -> vParallelAssembly/1
  NewModule_outputs/6 -> [vParallelAssembly1]
  [vCell1] -> vCellMux/1
  vCellMux/1 -> vCell/1
  NewModule_outputs/5 -> [vCell1]
  [socParallelAssembly1] -> socParallelAssemblyMux/1
  socParallelAssemblyMux/1 -> socParallelAssembly/1
  NewModule_outputs/4 -> [socParallelAssembly1]
  [socCell1] -> socCellMux/1
  socCellMux/1 -> socCell/1
  NewModule_outputs/3 -> [socCell1]
  [numCyclesCell1] -> numCyclesCellMux/1
  numCyclesCellMux/1 -> numCyclesCell/1
  NewModule_outputs/2 -> [numCyclesCell1]
  [iCell1] -> iCellMux/1
  iCellMux/1 -> iCell/1
  NewModule_outputs/1 -> [iCell1]
  connections:
  NewModule/RConn1 -- -/RConn1
  NewModule/LConn1 -- +/RConn1

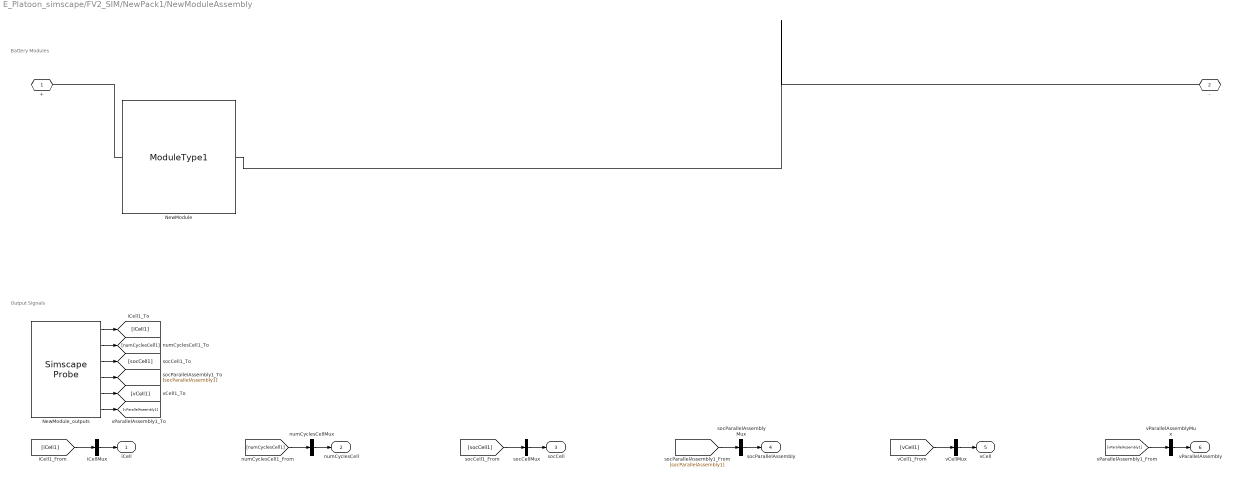
== system E_Platoon_simscape/FV2_SIM/NewPack1/NewModuleAssembly ==
  note: Output Signals
  note: Battery Modules
  NewModule : Batteries_lib/Modules/ModuleType1  SOC_vecCell=[0, .01, .02, .03, .04, .05, .06, .07, .08, .09, .1, .11, .12, .13, .14, .15, .16, .17, .18, .19, .2, .21, .22, .23, .24, .25, .26, .27, .28, .29, .3, .31, .32, .33, .34, .35, .36, .37, .38, .39, .4, .41, .42, .43, .44, .45, .46, .47, .48, .49, .5, .51, .52, .53, .54, .55, .56, .57, .58, .59, .6, .61, .62, .63, .64, .65, .66, .67, .68, .69, .7, .71, .72, .73, .74, .75, .76, .77, .78, .79, .8, .81, .82, .83, .84, .85, .86, .87, .88, .89, .9, .91, .92, .93, .94, .95, .96, .97, .98, .99, 1]  V0_vecCell=[35.84591, 36.10202, 36.35814, 36.61425, 36.87037, 37.12649, 37.3826, 37.63872, 37.89483, 38.09951, 38.20904, 38.28916, 38.37306, 38.42308, 38.45482, 38.47744, 38.49779, 38.54815, 38.5883, 38.63829, 38.68732, 38.72975, 38.77111, 38.80795, 38.83724, 38.8617, 38.89023, 38.9273, 38.96054, 38.98786, 39.01519, 39.03864, 39.06385, 39.08223, 39.1006, 39.11898, 39.13735, 39.15508, 39.16412, 39.17437, 39.18528, 39.19619, 39.20709, 39.21696, 39.22232, 39.22753, 39.23277, 39.23672, 39.23942, 39.24211, 39.24481, 39.24786, 39.25094, 39.2539, 39.25686, 39.26099, 39.26708, 39.27551, 39.28394, 39.29233, 39.30067, 39.31557, 39.33487, 39.35402, 39.37113, 39.38825, 39.40815, 39.43406, 39.46187, 39.48968, 39.51913, 39.55031, 39.5817, 39.60619, 39.62271, 39.63907, 39.65521, 39.67134, 39.68137, 39.69071, 39.70005, 39.7052, 39.70868, 39.70916, 39.70862, 39.70807, 39.70752, 39.71037, 39.72142, 39.72908, 39.73651, 39.73911, 39.73577, 39.72919, 39.73278, 39.7392, 39.74638, 39.75462, 39.8136, 40.01141, 40.30627] V  V_rangeCell=[27, Inf] V  R0_vecCell=[.47635, .41138, .35007, .29417, .24882, .2142, .18886, .17031, .1569, .14398, .13028, .11716, .10632, .09512, .08414, .07347, .06467, .05964, .05477, .05154, .04841, .04625, .04448, .04297, .04112, .03908, .0378, .03771, .03746, .03699, .03652, .03598, .03587, .03552, .03517, .03481, .03446, .03417, .03358, .03336, .03321, .03305, .0329, .0327, .03227, .03186, .03148, .03105, .03058, .03011, .02964, .02918, .02875, .02834, .02792, .02762, .02745, .02737, .02729, .02722, .02715, .0274, .02786, .0283, .02854, .02877, .02906, .02956, .03013, .0307, .03135, .03204, .03271, .03308, .03307, .03314, .03323, .03332, .03312, .03288, .03264, .03224, .03172, .03113, .03057, .03001, .02945, .02905, .02924, .0293, .02938, .02923, .02879, .02803, .02792, .02793, .02786, .02652, .02587, .02701, .00941] Ohm  AHCell=50.41 A*hr  extrapolation_optionCell=simscape.enum.extrapolation.nearest  P=18  S=18  iCell_specify=off  iCell_priority=None  iCell=0 A  iCell_nominal_specify=off  iCell_nominal_value=1  iCell_nominal_unit=A  vCell_specify=off  vCell_priority=None  vCell=0 V  vCell_nominal_specify=off  vCell_nominal_value=1  vCell_nominal_unit=V  socCell_specify=off  socCell_priority=High  socCell=1  socCell_nominal_specify=off  socCell_nominal_value=1  socCell_nominal_unit=1  numCyclesCell_specify=off  numCyclesCell_priority=High  numCyclesCell=0  numCyclesCell_nominal_specify=off  numCyclesCell_nominal_value=1  numCyclesCell_nominal_unit=1  vParallelAssembly_specify=off  vParallelAssembly_priority=None  vParallelAssembly=repmat(0, 18, 1) V  vParallelAssembly_nominal_specify=off  vParallelAssembly_nominal_value=1  vParallelAssembly_nominal_unit=V  socParallelAssembly_specify=off  socParallelAssembly_priority=None  socParallelAssembly=repmat(1, 18, 1)  socParallelAssembly_nominal_specify=off  socParallelAssembly_nominal_value=1  socParallelAssembly_nominal_unit=1
      settings: InternalSimscapePortConfiguration="{\"Bottom\":[{\"id\":\"n\",\"label\":\"-\",\"type\":\"foundation.electrical.electrical\"}],\"Left\":[],\"Right\":[],\"Top\":[{\"id\":\"p\",\"label\":\"+\",\"type\":\"foundation.electrical.electrical\"}]}"
  NewModule_outputs : SimscapeProbe  BoundBlock=11219  Variables="{\"iCell\":{\"Unit\":\"A\",\"PortLabel\":\"iCell\",\"Probing\":\"ON\"},\"numCyclesCell\":{\"Unit\":\"1\",\"PortLabel\":\"numCyclesCell\",\"Probing\":\"ON\"},\"socCell\":{\"Unit\":\"1\",\"PortLabel\":\"socCell\",\"Probing\":\"ON\"},\"socParallelAssembly\":{\"Unit\":\"1\",\"PortLabel\":\"socParallelAssembly\",\"Probing\":\"ON\"},\"vCell\":{\"Unit\":\"V\",\"PortLabel\":\"vCell\",\"Probing\":\"ON\"},\"vParallelAssembly\":{\"Unit\":\"V\",\"PortLabel\":\"vParallelAssembly\",\"Probing\":\"ON\"}}"
  iCellMux : Mux  Inputs=1
  numCyclesCellMux : Mux  Inputs=1
  socCellMux : Mux  Inputs=1
  socParallelAssemblyMux : Mux  Inputs=1
  vCellMux : Mux  Inputs=1
  vParallelAssemblyMux : Mux  Inputs=1
  + : PMIOPort  Side=Left
  - : PMIOPort  Port=2  Side=Right
  iCell : Outport
  numCyclesCell : Outport  Port=2
  socCell : Outport  Port=3
  socParallelAssembly : Outport  Port=4
  vCell : Outport  Port=5
  vParallelAssembly : Outport  Port=6
  wires:
  [vParallelAssembly1] -> vParallelAssemblyMux/1
  vParallelAssemblyMux/1 -> vParallelAssembly/1
  NewModule_outputs/6 -> [vParallelAssembly1]
  [vCell1] -> vCellMux/1
  vCellMux/1 -> vCell/1
  NewModule_outputs/5 -> [vCell1]
  [socParallelAssembly1] -> socParallelAssemblyMux/1
  socParallelAssemblyMux/1 -> socParallelAssembly/1
  NewModule_outputs/4 -> [socParallelAssembly1]
  [socCell1] -> socCellMux/1
  socCellMux/1 -> socCell/1
  NewModule_outputs/3 -> [socCell1]
  [numCyclesCell1] -> numCyclesCellMux/1
  numCyclesCellMux/1 -> numCyclesCell/1
  NewModule_outputs/2 -> [numCyclesCell1]
  [iCell1] -> iCellMux/1
  iCellMux/1 -> iCell/1
  NewModule_outputs/1 -> [iCell1]
  connections:
  NewModule/RConn1 -- -/RConn1
  NewModule/LConn1 -- +/RConn1

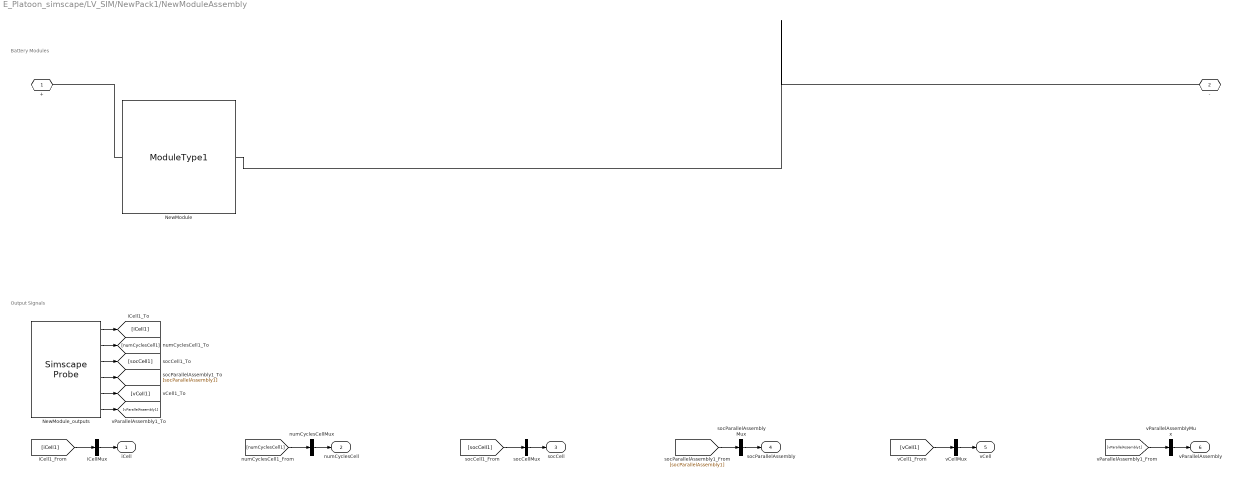
== system E_Platoon_simscape/LV_SIM/NewPack1/NewModuleAssembly ==
  note: Output Signals
  note: Battery Modules
  NewModule : Batteries_lib/Modules/ModuleType1  SOC_vecCell=[0, .01, .02, .03, .04, .05, .06, .07, .08, .09, .1, .11, .12, .13, .14, .15, .16, .17, .18, .19, .2, .21, .22, .23, .24, .25, .26, .27, .28, .29, .3, .31, .32, .33, .34, .35, .36, .37, .38, .39, .4, .41, .42, .43, .44, .45, .46, .47, .48, .49, .5, .51, .52, .53, .54, .55, .56, .57, .58, .59, .6, .61, .62, .63, .64, .65, .66, .67, .68, .69, .7, .71, .72, .73, .74, .75, .76, .77, .78, .79, .8, .81, .82, .83, .84, .85, .86, .87, .88, .89, .9, .91, .92, .93, .94, .95, .96, .97, .98, .99, 1]  V0_vecCell=[35.84591, 36.10202, 36.35814, 36.61425, 36.87037, 37.12649, 37.3826, 37.63872, 37.89483, 38.09951, 38.20904, 38.28916, 38.37306, 38.42308, 38.45482, 38.47744, 38.49779, 38.54815, 38.5883, 38.63829, 38.68732, 38.72975, 38.77111, 38.80795, 38.83724, 38.8617, 38.89023, 38.9273, 38.96054, 38.98786, 39.01519, 39.03864, 39.06385, 39.08223, 39.1006, 39.11898, 39.13735, 39.15508, 39.16412, 39.17437, 39.18528, 39.19619, 39.20709, 39.21696, 39.22232, 39.22753, 39.23277, 39.23672, 39.23942, 39.24211, 39.24481, 39.24786, 39.25094, 39.2539, 39.25686, 39.26099, 39.26708, 39.27551, 39.28394, 39.29233, 39.30067, 39.31557, 39.33487, 39.35402, 39.37113, 39.38825, 39.40815, 39.43406, 39.46187, 39.48968, 39.51913, 39.55031, 39.5817, 39.60619, 39.62271, 39.63907, 39.65521, 39.67134, 39.68137, 39.69071, 39.70005, 39.7052, 39.70868, 39.70916, 39.70862, 39.70807, 39.70752, 39.71037, 39.72142, 39.72908, 39.73651, 39.73911, 39.73577, 39.72919, 39.73278, 39.7392, 39.74638, 39.75462, 39.8136, 40.01141, 40.30627] V  V_rangeCell=[27, Inf] V  R0_vecCell=[.47635, .41138, .35007, .29417, .24882, .2142, .18886, .17031, .1569, .14398, .13028, .11716, .10632, .09512, .08414, .07347, .06467, .05964, .05477, .05154, .04841, .04625, .04448, .04297, .04112, .03908, .0378, .03771, .03746, .03699, .03652, .03598, .03587, .03552, .03517, .03481, .03446, .03417, .03358, .03336, .03321, .03305, .0329, .0327, .03227, .03186, .03148, .03105, .03058, .03011, .02964, .02918, .02875, .02834, .02792, .02762, .02745, .02737, .02729, .02722, .02715, .0274, .02786, .0283, .02854, .02877, .02906, .02956, .03013, .0307, .03135, .03204, .03271, .03308, .03307, .03314, .03323, .03332, .03312, .03288, .03264, .03224, .03172, .03113, .03057, .03001, .02945, .02905, .02924, .0293, .02938, .02923, .02879, .02803, .02792, .02793, .02786, .02652, .02587, .02701, .00941] Ohm  AHCell=50.41 A*hr  extrapolation_optionCell=simscape.enum.extrapolation.nearest  P=18  S=18  iCell_specify=off  iCell_priority=None  iCell=0 A  iCell_nominal_specify=off  iCell_nominal_value=1  iCell_nominal_unit=A  vCell_specify=off  vCell_priority=None  vCell=0 V  vCell_nominal_specify=off  vCell_nominal_value=1  vCell_nominal_unit=V  socCell_specify=off  socCell_priority=High  socCell=1  socCell_nominal_specify=off  socCell_nominal_value=1  socCell_nominal_unit=1  numCyclesCell_specify=off  numCyclesCell_priority=High  numCyclesCell=0  numCyclesCell_nominal_specify=off  numCyclesCell_nominal_value=1  numCyclesCell_nominal_unit=1  vParallelAssembly_specify=off  vParallelAssembly_priority=None  vParallelAssembly=repmat(0, 18, 1) V  vParallelAssembly_nominal_specify=off  vParallelAssembly_nominal_value=1  vParallelAssembly_nominal_unit=V  socParallelAssembly_specify=off  socParallelAssembly_priority=None  socParallelAssembly=repmat(1, 18, 1)  socParallelAssembly_nominal_specify=off  socParallelAssembly_nominal_value=1  socParallelAssembly_nominal_unit=1
      settings: InternalSimscapePortConfiguration="{\"Bottom\":[{\"id\":\"n\",\"label\":\"-\",\"type\":\"foundation.electrical.electrical\"}],\"Left\":[],\"Right\":[],\"Top\":[{\"id\":\"p\",\"label\":\"+\",\"type\":\"foundation.electrical.electrical\"}]}"
  NewModule_outputs : SimscapeProbe  BoundBlock=11059  Variables="{\"iCell\":{\"Unit\":\"A\",\"PortLabel\":\"iCell\",\"Probing\":\"ON\"},\"numCyclesCell\":{\"Unit\":\"1\",\"PortLabel\":\"numCyclesCell\",\"Probing\":\"ON\"},\"socCell\":{\"Unit\":\"1\",\"PortLabel\":\"socCell\",\"Probing\":\"ON\"},\"socParallelAssembly\":{\"Unit\":\"1\",\"PortLabel\":\"socParallelAssembly\",\"Probing\":\"ON\"},\"vCell\":{\"Unit\":\"V\",\"PortLabel\":\"vCell\",\"Probing\":\"ON\"},\"vParallelAssembly\":{\"Unit\":\"V\",\"PortLabel\":\"vParallelAssembly\",\"Probing\":\"ON\"}}"
  iCellMux : Mux  Inputs=1
  numCyclesCellMux : Mux  Inputs=1
  socCellMux : Mux  Inputs=1
  socParallelAssemblyMux : Mux  Inputs=1
  vCellMux : Mux  Inputs=1
  vParallelAssemblyMux : Mux  Inputs=1
  + : PMIOPort  Side=Left
  - : PMIOPort  Port=2  Side=Right
  iCell : Outport
  numCyclesCell : Outport  Port=2
  socCell : Outport  Port=3
  socParallelAssembly : Outport  Port=4
  vCell : Outport  Port=5
  vParallelAssembly : Outport  Port=6
  wires:
  [vParallelAssembly1] -> vParallelAssemblyMux/1
  vParallelAssemblyMux/1 -> vParallelAssembly/1
  NewModule_outputs/6 -> [vParallelAssembly1]
  [vCell1] -> vCellMux/1
  vCellMux/1 -> vCell/1
  NewModule_outputs/5 -> [vCell1]
  [socParallelAssembly1] -> socParallelAssemblyMux/1
  socParallelAssemblyMux/1 -> socParallelAssembly/1
  NewModule_outputs/4 -> [socParallelAssembly1]
  [socCell1] -> socCellMux/1
  socCellMux/1 -> socCell/1
  NewModule_outputs/3 -> [socCell1]
  [numCyclesCell1] -> numCyclesCellMux/1
  numCyclesCellMux/1 -> numCyclesCell/1
  NewModule_outputs/2 -> [numCyclesCell1]
  [iCell1] -> iCellMux/1
  iCellMux/1 -> iCell/1
  NewModule_outputs/1 -> [iCell1]
  connections:
  NewModule/RConn1 -- -/RConn1
  NewModule/LConn1 -- +/RConn1
